simulink model "halozat_4_szet"  (R2013a)
settings: Solver=ode23s  StartTime=0.0  StopTime=5  MaxStep=0.0001  RelTol=1e-4
InitFcn:
  | punct
undefined symbols (not defined in the file or in its folder): get, Ion, Lithium
libraries: powerlib x79, simulink x37, dspsigops x18, powerlib_extras x4, dspsnks4 x2, dsparch4 x2, dspxfrm3 x1, commsequence2 x1, electricdrivelib x1
settings Model: ExtModeAutoUpdateStatusClock=off  Creator=gorbep  LastModifiedBy=Neukirchner László
settings SolverCC: PositivePriorityOrder=on
settings DataIOCC: SignalLoggingSaveFormat=ModelDataLogs
settings OptimizationCC: ExpressionDepthLimit=2147483647  InitFltsAndDblsToZero=on
settings DebuggingCC: MultiTaskDSMMsg=warning  MultiTaskCondExecSysMsg=none  FcnCallInpInsideContextMsg=UseLocalSettings  StrictBusMsg=None
settings RTWCC: IncludeERTFirstTime=on
settings GRTTargetCC: CodeReplacementLibrary=None  CombineOutputUpdateFcns=off  CPPClassGenCompliant=on  GRTInterface=on

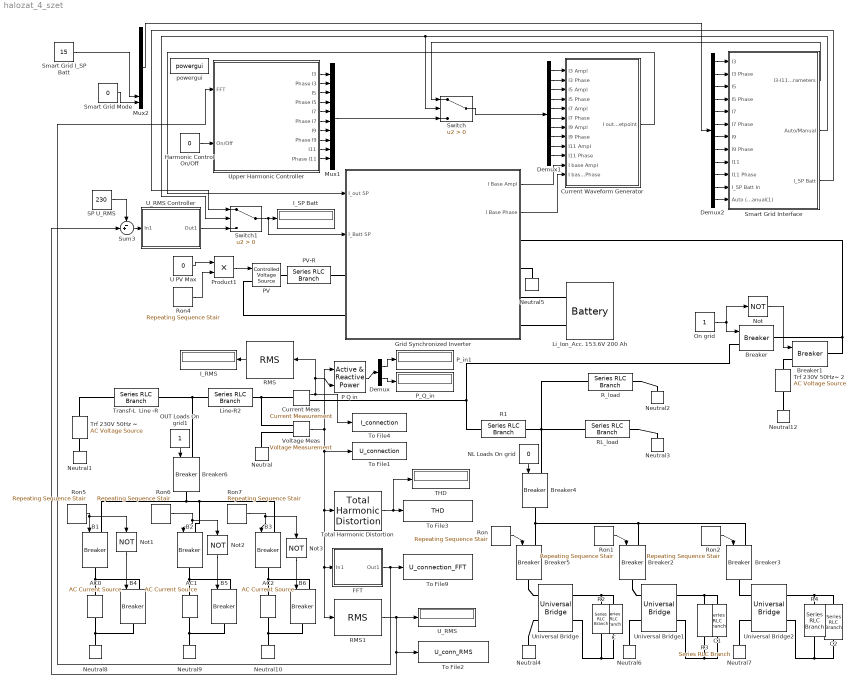
== system halozat_4_szet ==
  AC0 : powerlib/Electrical Sources/AC Current Source  Amplitude=-50  Phase=0  Frequency=50  SampleTime=0  Measurements=None
  AC1 : powerlib/Electrical Sources/AC Current Source  Amplitude=20  Phase=0  Frequency=50  SampleTime=0  Measurements=None
  AC2 : powerlib/Electrical Sources/AC Current Source  Amplitude=-30  Phase=0  Frequency=50  SampleTime=0  Measurements=None
  B{1..6} (6 alike) : powerlib/Elements/Breaker  BreakerResistance=0.01  InitialState=0  SnubberResistance=1e7  SnubberCapacitance=inf  SwitchingTimes="[ 1/60  5/60 ]"  External=on  Measurements=None  MoreParameters=off  NoBreakLoop=off
  Breaker{,1..6} (7 alike) : powerlib/Elements/Breaker  BreakerResistance=0.01  InitialState=0  SnubberResistance=1e7  SnubberCapacitance=inf  SwitchingTimes="[ 1/60  5/60 ]"  External=on  Measurements=None  MoreParameters=off  NoBreakLoop=off
  C : powerlib/Elements/Series RLC Branch  LConnTagsString=__new0  RConnTagsString=__new0  BranchType=C  Resistance=35.35  Inductance=0.1125  SetiL0=off  InitialCurrent=0  Capacitance=10e-3  Setx0=off  InitialVoltage=0  Measurements=None
  C1 : powerlib/Elements/Series RLC Branch  LConnTagsString=__new0  RConnTagsString=__new0  BranchType=C  Resistance=35.35  Inductance=0.1125  SetiL0=off  InitialCurrent=0  Capacitance=5e-3  Setx0=off  InitialVoltage=0  Measurements=None
  C2 : powerlib/Elements/Series RLC Branch  LConnTagsString=__new0  RConnTagsString=__new0  BranchType=C  Resistance=35.35  Inductance=0.1125  SetiL0=off  InitialCurrent=0  Capacitance=7e-3  Setx0=off  InitialVoltage=0  Measurements=None
  Current Meas : powerlib/Measurements/Current Measurement  PhasorSimulation=off  OutputType=Complex  PSBequivalent=0
  Current Waveform Generator : Subsystem
  Demux : Demux  Outputs=2
  Demux1 : Demux  Outputs=10
  Demux2 : Demux  Outputs=12
  FFT : Subsystem
  Grid Synchronized Inverter : Subsystem
  Harmonic Control On/Off : Constant  Value=0
  I_RMS : Display
  I_SP Batt : Display
  Li_Ion_Acc. 153.6V 200 Ah : electricdrivelib/Extra Sources/Battery  BatType=Lithium-Ion  ShowDetailedParameters=off  NomV=153.6  NomQ=200  SOC=100  PresetModel=off  MaxQ=210  FullV=274.6189824  Dis_rate=173.913  R=0.00768  Normal_OP=361.7392  expZone=[254.8950528 19.652174]  Dis_Char=off  current=[1.5 3]  Units=Ampere-hour  Batt_Tr=30
  Line-R2 : powerlib/Elements/Series RLC Branch  LConnTagsString=__new0  RConnTagsString=__new0  BranchType=R  Resistance=0.1  Inductance=0.003185  SetiL0=off  InitialCurrent=0  Capacitance=1.0  Setx0=off  InitialVoltage=0  Measurements=None
  Mux1 : Mux  Inputs=10
  Mux2 : Mux  Inputs=12
  NL Loads On grid : Constant  Value=0
  Neutral{,1..10,12} (12 alike) : powerlib/Elements/Neutral  LConnTagsString=a  NodeNumber=10
  Not{,1..3} (4 alike) : Logic  Operator=NOT  IconShape=distinctive  AllPortsSameDT=off  OutDataTypeStr=boolean
  OUT Loads On grid1 : Constant
  On grid : Constant
  P Q in : powerlib_extras/Measurements/Active & Reactive Power  f1=50
  PV : powerlib/Electrical Sources/Controlled Voltage Source  Initialize=off  Source_Type=AC  Amplitude=0  Phase=0  Frequency=0  Measurements=None
  PV-R : powerlib/Elements/Series RLC Branch  LConnTagsString=__new0  RConnTagsString=__new0  BranchType=R  Resistance=5  Inductance=0.1  SetiL0=off  InitialCurrent=0  Capacitance=1.0  Setx0=off  InitialVoltage=0  Measurements=None
  P_Q_in : Display
  P_in1 : Display
  Product1 : Product  RndMeth=Zero
  R1 : powerlib/Elements/Series RLC Branch  LConnTagsString=__new0  RConnTagsString=__new0  BranchType=R  Resistance=0.2  Inductance=0.003185  SetiL0=off  InitialCurrent=0  Capacitance=1.0  Setx0=off  InitialVoltage=0  Measurements=None
  R2 : powerlib/Elements/Series RLC Branch  LConnTagsString=__new0  RConnTagsString=__new0  BranchType=R  Resistance=25  Inductance=0.003185  SetiL0=off  InitialCurrent=0  Capacitance=1.0  Setx0=off  InitialVoltage=0  Measurements=None
  R3 : powerlib/Elements/Series RLC Branch  LConnTagsString=__new0  RConnTagsString=__new0  BranchType=R  Resistance=50  Inductance=0.003185  SetiL0=off  InitialCurrent=0  Capacitance=1.0  Setx0=off  InitialVoltage=0  Measurements=None
  R4 : powerlib/Elements/Series RLC Branch  LConnTagsString=__new0  RConnTagsString=__new0  BranchType=R  Resistance=35  Inductance=0.003185  SetiL0=off  InitialCurrent=0  Capacitance=1.0  Setx0=off  InitialVoltage=0  Measurements=None
  RL_load : powerlib/Elements/Series RLC Branch  LConnTagsString=__new0  RConnTagsString=__new0  BranchType=RL  Resistance=35.35  Inductance=0.1125  SetiL0=off  InitialCurrent=0  Capacitance=1.0  Setx0=off  InitialVoltage=0  Measurements=None
  RMS : powerlib_extras/Measurements/RMS  f1=50
  RMS1 : powerlib_extras/Measurements/RMS  f1=50
  R_load : powerlib/Elements/Series RLC Branch  LConnTagsString=__new0  RConnTagsString=__new0  BranchType=R  Resistance=50  Inductance=0.003185  SetiL0=off  InitialCurrent=0  Capacitance=1.0  Setx0=off  InitialVoltage=0  Measurements=None
  Ron : simulink/Sources/Repeating Sequence Stair  OutValues=[1 1 0 0 0 0 0 0 0 0].'  tsamp=10  OutMin=[]  OutMax=[]  OutDataTypeStr=float('double')  OutputDataTypeScalingMode=Specify via dialog  OutDataType=float('double')  ConRadixGroup=Best Precision: Vector-wise  OutScaling=2^-12
  Ron1 : simulink/Sources/Repeating Sequence Stair  OutValues=[0 0 0 1 1 0 0 0 0 0].'  tsamp=10  OutMin=[]  OutMax=[]  OutDataTypeStr=float('double')  OutputDataTypeScalingMode=Specify via dialog  OutDataType=float('double')  ConRadixGroup=Best Precision: Vector-wise  OutScaling=2^-12
  Ron2 : simulink/Sources/Repeating Sequence Stair  OutValues=[0 0 0 0 1 0 0 0 0 0].'  tsamp=10  OutMin=[]  OutMax=[]  OutDataTypeStr=float('double')  OutputDataTypeScalingMode=Specify via dialog  OutDataType=float('double')  ConRadixGroup=Best Precision: Vector-wise  OutScaling=2^-12
  Ron4 : simulink/Sources/Repeating Sequence Stair  OutValues=[1 1 0 0].'  tsamp=0.5  OutMin=[]  OutMax=[]  OutDataTypeStr=float('double')  OutputDataTypeScalingMode=Specify via dialog  OutDataType=float('double')  ConRadixGroup=Best Precision: Vector-wise  OutScaling=2^-12
  Ron5 : simulink/Sources/Repeating Sequence Stair  OutValues=[0 1 0 0 0 0 0 0 0 0].'  tsamp=1  OutMin=[]  OutMax=[]  OutDataTypeStr=float('double')  OutputDataTypeScalingMode=Specify via dialog  OutDataType=float('double')  ConRadixGroup=Best Precision: Vector-wise  OutScaling=2^-12
  Ron6 : simulink/Sources/Repeating Sequence Stair  OutValues="[0 0 0  1 0 0 0 0 0 0].'"  tsamp=1  OutMin=[]  OutMax=[]  OutDataTypeStr=float('double')  OutputDataTypeScalingMode=Specify via dialog  OutDataType=float('double')  ConRadixGroup=Best Precision: Vector-wise  OutScaling=2^-12
  Ron7 : simulink/Sources/Repeating Sequence Stair  OutValues=[0 0 0 0 1 0 0 0 0 0].'  tsamp=1  OutMin=[]  OutMax=[]  OutDataTypeStr=float('double')  OutputDataTypeScalingMode=Specify via dialog  OutDataType=float('double')  ConRadixGroup=Best Precision: Vector-wise  OutScaling=2^-12
  SP U_RMS : Constant  Value=230
  Smart Grid I_SP Batt : Constant  Value=15
  Smart Grid Mode : Constant  Value=0
  Smart Grid Interface : Subsystem
  Sum3 : Sum  Inputs=-+|
  Switch : Switch  Criteria=u2 > Threshold
  Switch1 : Switch  Criteria=u2 > Threshold
  THD : Display
  To File1 : ToFile  Filename=U_connection  MatrixName=y  SampleTime=5e-5
  To File2 : ToFile  Filename=U_conn_RMS  MatrixName=y  SampleTime=1e-3
  To File3 : ToFile  Filename=THD  MatrixName=y  SampleTime=1e-3
  To File4 : ToFile  Filename=I_connection  MatrixName=y  SampleTime=5e-5
  To File9 : ToFile  Filename=U_connection_FFT  MatrixName=y  SampleTime=1e-3
  Total Harmonic Distortion : powerlib_extras/Measurements/Total Harmonic Distortion  f1=50
  Transf-L  Line -R : powerlib/Elements/Series RLC Branch  LConnTagsString=__new0  RConnTagsString=__new0  BranchType=RL  Resistance=0.4  Inductance=0.003185  SetiL0=off  InitialCurrent=0  Capacitance=1.0  Setx0=off  InitialVoltage=0  Measurements=None
  Trf 230V 50Hz ~ : powerlib/Electrical Sources/AC Voltage Source  Amplitude=325.2691  Phase=0  Frequency=50  SampleTime=0  Measurements=None
  Trf 230V 50Hz~ 2 : powerlib/Electrical Sources/AC Voltage Source  Amplitude=325.2691  Phase=0  Frequency=50  SampleTime=0  Measurements=None
  U PV Max : Constant  Value=0
  U_RMS : Display
  U_RMS Controller : Subsystem
  Universal Bridge : powerlib/Power Electronics/Universal Bridge  Arms=2  SnubberResistance=1e5  SnubberCapacitance=inf  Device=Diodes  Ron=1e-3  Lon=0  ForwardVoltages="[  0  0  ]"  ForwardVoltage=0.8  GTOparameters=[ 10e-6 , 20e-6 ]  IGBTparameters=[ 1e-6 , 2e-6 ]  Measurements=None  Measurements_2=None  converterType=Rectifier
  Universal Bridge1 : powerlib/Power Electronics/Universal Bridge  Arms=2  SnubberResistance=1e5  SnubberCapacitance=inf  Device=Diodes  Ron=1e-3  Lon=0  ForwardVoltages="[  0  0  ]"  ForwardVoltage=0.8  GTOparameters=[ 10e-6 , 20e-6 ]  IGBTparameters=[ 1e-6 , 2e-6 ]  Measurements=None  Measurements_2=None  converterType=Rectifier
  Universal Bridge2 : powerlib/Power Electronics/Universal Bridge  Arms=2  SnubberResistance=1e5  SnubberCapacitance=inf  Device=Diodes  Ron=1e-3  Lon=0  ForwardVoltages="[  0  0  ]"  ForwardVoltage=0.8  GTOparameters=[ 10e-6 , 20e-6 ]  IGBTparameters=[ 1e-6 , 2e-6 ]  Measurements=None  Measurements_2=None  converterType=Rectifier
  Upper Harmonic Controller : Subsystem
  Voltage Meas : powerlib/Measurements/Voltage Measurement  PhasorSimulation=off  OutputType=Complex  PSBequivalent=0
  powergui : powerlib/powergui  SimulationMode=Continuous  SolverType=Tustin  SampleTime=50e-6  frequency=60  SPID=off  DisableSnubberDevices=off  DisableRonSwitches=off  DisableVfSwitches=off  SwTol=0  Interpol=off  DisplayEquations=off  frequencyindice=50  Pbase=100e6  ErrMax=1e-4  Iterations=50  UnitsV=kV  UnitsW=MW  FunctionMessages=off  echomessages=off  HookPort=off  EnableUseOfTLC=off  x0status=blocks  RestoreLinks=warning  ResistiveCurrentMeasurement=off  Frange=[0:2:500]  Ylog=off  Xlog=on  ShowGrid=off  save=off  variable=ZData  structure=0  ZoomFFT=on  StartTime=0.0  cycles=1  DisplayStyle=1  fundamental=60  FreqAxis=off  MaxFrequency=1000  frequencyindicesteady=1  RmsSteady=1  display=off  Ts=0  methode=off
  wires:
  Voltage Meas/1 -> To File1/1, Total Harmonic Distortion/1, RMS1/1, FFT/1(In1), P Q in/1
  Current Meas/1 -> To File4/1, RMS/1, P Q in/2
  On grid/1 -> Breaker/1, Not/1
  Not/1 -> Breaker1/1
  Total Harmonic Distortion/1 -> THD/1, To File3/1
  Harmonic Control On/Off/1 -> Upper Harmonic Controller/2(On/Off)
  FFT/1(Out1) -> Upper Harmonic Controller/1(FFT), To File9/1
  Ron1/1 -> Breaker2/1
  Grid Synchronized Inverter/2(I Base Phase) -> Current Waveform Generator/12(I base Phase)
  Current Waveform Generator/1(I out Setpoint) -> Grid Synchronized Inverter/1(I_out SP)
  Ron/1 -> Breaker5/1
  RMS/1 -> I_RMS/1
  Demux/1 -> P_in1/1
  P Q in/1 -> Demux/1
  Demux/2 -> P_Q_in/1
  Product1/1 -> PV/1
  U PV Max/1 -> Product1/1
  Ron4/1 -> Product1/2
  RMS1/1 -> U_RMS/1, Sum3/2, To File2/1
  Ron2/1 -> Breaker3/1
  NL Loads On grid/1 -> Breaker4/1
  OUT Loads On grid1/1 -> Breaker6/1
  Sum3/1 -> U_RMS Controller/1(In1)
  SP U_RMS/1 -> Sum3/1
  Ron5/1 -> B1/1, Not1/1
  Ron6/1 -> B2/1, Not2/1
  Ron7/1 -> B3/1, Not3/1
  Not1/1 -> B4/1
  Not2/1 -> B5/1
  Not3/1 -> B6/1
  Upper Harmonic Controller/1(I3) -> Mux1/1
  Upper Harmonic Controller/2(Phase I3) -> Mux1/2
  Upper Harmonic Controller/3(I5) -> Mux1/3
  Upper Harmonic Controller/4(Phase I5) -> Mux1/4
  Upper Harmonic Controller/5(I7) -> Mux1/5
  Upper Harmonic Controller/6(Phase I7) -> Mux1/6
  Upper Harmonic Controller/7(I9) -> Mux1/7
  Upper Harmonic Controller/8(Phase I9) -> Mux1/8
  Upper Harmonic Controller/9(I11) -> Mux1/9
  Upper Harmonic Controller/10(Phase I11) -> Mux1/10
  Demux1/1 -> Current Waveform Generator/1(I3 Ampl)
  Demux1/2 -> Current Waveform Generator/2(I3 Phase)
  Demux1/3 -> Current Waveform Generator/3(I5 Ampl)
  Demux1/4 -> Current Waveform Generator/4(I5 Phase)
  Demux1/5 -> Current Waveform Generator/5(I7 Ampl)
  Demux1/6 -> Current Waveform Generator/6(I7 Phase)
  Demux1/7 -> Current Waveform Generator/7(I9 Ampl)
  Demux1/8 -> Current Waveform Generator/8(I9 Phase)
  Demux1/9 -> Current Waveform Generator/9(I11 Ampl)
  Demux1/10 -> Current Waveform Generator/10(I11 Phase)
  Switch/1 -> Demux1/1
  Mux1/1 -> Switch/3
  Smart Grid Interface/1(I3-I11 Parameters) -> Switch/1
  Smart Grid Interface/2(Auto/Manual) -> Switch/2, Switch1/2
  U_RMS Controller/1(Out1) -> Switch1/3
  Switch1/1 -> I_SP Batt/1, Grid Synchronized Inverter/2(I_Batt SP)
  Smart Grid Interface/3(I_SP Batt) -> Switch1/1
  Grid Synchronized Inverter/1(I Base Ampl) -> Current Waveform Generator/11(I base Ampl)
  Demux2/1 -> Smart Grid Interface/1(I3)
  Demux2/2 -> Smart Grid Interface/2(I3 Phase)
  Demux2/3 -> Smart Grid Interface/3(I5)
  Demux2/4 -> Smart Grid Interface/4(I5 Phase)
  Demux2/5 -> Smart Grid Interface/5(I7)
  Demux2/6 -> Smart Grid Interface/6(I7 Phase)
  Demux2/7 -> Smart Grid Interface/7(I9)
  Demux2/8 -> Smart Grid Interface/8(I9 Phase)
  Demux2/9 -> Smart Grid Interface/9(I11)
  Demux2/10 -> Smart Grid Interface/10(I11 Phase)
  Demux2/11 -> Smart Grid Interface/11(I_SP Batt In)
  Demux2/12 -> Smart Grid Interface/12(Auto (0) / Manual(1))
  Mux2/1 -> Demux2/1
  Smart Grid Mode/1 -> Mux2/12
  Smart Grid I_SP Batt/1 -> Mux2/11
  connections:
  Trf 230V 50Hz ~/LConn1 -- Neutral1/LConn1
  Transf-L  Line -R/LConn1 -- Trf 230V 50Hz ~/RConn1
  Voltage Meas/LConn1 -- Current Meas/LConn1 -- Line-R2/RConn1
  Neutral/LConn1 -- Voltage Meas/LConn2
  Current Meas/RConn1 -- R1/LConn1 -- Breaker/LConn1
  R_load/RConn1 -- Neutral2/LConn1
  RL_load/RConn1 -- Neutral3/LConn1
  Neutral4/LConn1 -- Universal Bridge/LConn2
  Trf 230V 50Hz~ 2/LConn1 -- Neutral12/LConn1
  Grid Synchronized Inverter/RConn1 -- Breaker1/RConn1 -- Breaker/RConn1
  Breaker2/LConn1 -- Breaker3/LConn1 -- Breaker5/LConn1 -- Breaker4/RConn1
  Breaker1/LConn1 -- Trf 230V 50Hz~ 2/RConn1
  Breaker5/RConn1 -- Universal Bridge/LConn1
  C/LConn1 -- Universal Bridge/RConn1 -- R2/LConn1
  C/RConn1 -- Universal Bridge/RConn2 -- R2/RConn1
  Universal Bridge1/RConn1 -- C1/LConn1 -- R3/LConn1
  Breaker2/RConn1 -- Universal Bridge1/LConn1
  Neutral6/LConn1 -- Universal Bridge1/LConn2
  PV/RConn1 -- PV-R/LConn1
  PV/LConn1 -- Grid Synchronized Inverter/LConn2
  PV-R/RConn1 -- Grid Synchronized Inverter/LConn1
  Neutral5/LConn1 -- Grid Synchronized Inverter/RConn2
  Universal Bridge1/RConn2 -- C1/RConn1 -- R3/RConn1
  Grid Synchronized Inverter/RConn3 -- Li_Ion_Acc. 153.6V 200 Ah/LConn1
  Grid Synchronized Inverter/RConn4 -- Li_Ion_Acc. 153.6V 200 Ah/LConn2
  Line-R2/LConn1 -- Transf-L  Line -R/RConn1 -- Breaker6/LConn1
  R4/LConn1 -- Universal Bridge2/RConn1 -- C2/LConn1
  R4/RConn1 -- Universal Bridge2/RConn2 -- C2/RConn1
  Breaker3/RConn1 -- Universal Bridge2/LConn1
  Neutral7/LConn1 -- Universal Bridge2/LConn2
  AC0/LConn1 -- Neutral8/LConn1 -- B4/RConn1
  B1/RConn1 -- AC0/RConn1 -- B4/LConn1
  B2/RConn1 -- AC1/RConn1 -- B5/LConn1
  AC1/LConn1 -- Neutral9/LConn1 -- B5/RConn1
  B3/RConn1 -- AC2/RConn1 -- B6/LConn1
  AC2/LConn1 -- Neutral10/LConn1 -- B6/RConn1
  R1/RConn1 -- RL_load/LConn1 -- R_load/LConn1 -- Breaker4/LConn1
  B2/LConn1 -- B3/LConn1 -- B1/LConn1 -- Breaker6/RConn1

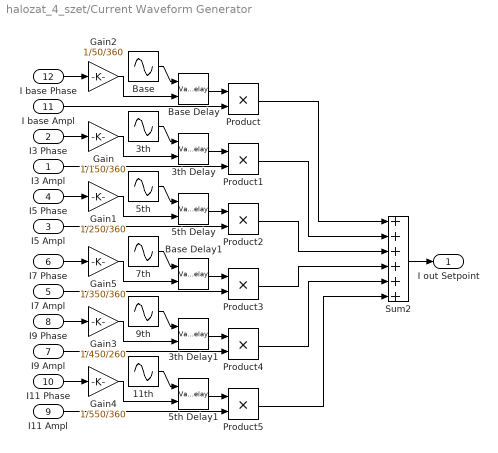
== system halozat_4_szet/Current Waveform Generator ==
  I3 Ampl : Inport
  I3 Phase : Inport  Port=2
  I5 Ampl : Inport  Port=3
  I5 Phase : Inport  Port=4
  I7 Ampl : Inport  Port=5
  I7 Phase : Inport  Port=6
  I9 Ampl : Inport  Port=7
  I9 Phase : Inport  Port=8
  I11 Ampl : Inport  Port=9
  I11 Phase : Inport  Port=10
  I base Ampl : Inport  Port=11
  I base Phase : Inport  Port=12
  11th : Sin  Frequency=110*pi  SampleTime=0
  3th : Sin  Frequency=300*pi  SampleTime=0
  3th Delay : VariableTransportDelay  MaximumDelay=10  ZeroDelay=on
  3th Delay1 : VariableTransportDelay  MaximumDelay=10  ZeroDelay=on
  5th : Sin  Frequency=500*pi  SampleTime=0
  5th Delay : VariableTransportDelay  MaximumDelay=10  ZeroDelay=on
  5th Delay1 : VariableTransportDelay  MaximumDelay=10  ZeroDelay=on
  7th : Sin  Frequency=700*pi  SampleTime=0
  9th : Sin  Frequency=900*pi  SampleTime=0
  Base : Sin  Frequency=100*pi  SampleTime=0
  Base Delay : VariableTransportDelay  MaximumDelay=10  ZeroDelay=on
  Base Delay1 : VariableTransportDelay  MaximumDelay=10  ZeroDelay=on
  Gain : Gain  Gain=1/150/360
  Gain1 : Gain  Gain=1/250/360
  Gain2 : Gain  Gain=1/50/360
  Gain3 : Gain  Gain=1/450/260
  Gain4 : Gain  Gain=1/550/360
  Gain5 : Gain  Gain=1/350/360
  Product{,1..5} (6 alike) : Product  RndMeth=Zero
  Sum2 : Sum  Inputs=++++++
  I out Setpoint : Outport
  wires:
  Base/1 -> Base Delay/1
  Base Delay/1 -> Product/1
  3th Delay/1 -> Product1/1
  5th Delay/1 -> Product2/1
  3th/1 -> 3th Delay/1
  5th/1 -> 5th Delay/1
  Gain/1 -> 3th Delay/2
  Gain1/1 -> 5th Delay/2
  Gain2/1 -> Base Delay/2
  I base Ampl/1 -> Product/2
  I base Phase/1 -> Gain2/1
  I3 Phase/1 -> Gain/1
  Sum2/1 -> I out Setpoint/1
  I3 Ampl/1 -> Product1/2
  I5 Phase/1 -> Gain1/1
  I5 Ampl/1 -> Product2/2
  7th/1 -> Base Delay1/1
  Base Delay1/1 -> Product3/1
  3th Delay1/1 -> Product4/1
  5th Delay1/1 -> Product5/1
  9th/1 -> 3th Delay1/1
  11th/1 -> 5th Delay1/1
  Gain3/1 -> 3th Delay1/2
  Gain4/1 -> 5th Delay1/2
  Gain5/1 -> Base Delay1/2
  I7 Ampl/1 -> Product3/2
  I7 Phase/1 -> Gain5/1
  I9 Phase/1 -> Gain3/1
  I9 Ampl/1 -> Product4/2
  I11 Phase/1 -> Gain4/1
  I11 Ampl/1 -> Product5/2
  Product/1 -> Sum2/1
  Product1/1 -> Sum2/2
  Product2/1 -> Sum2/3
  Product3/1 -> Sum2/4
  Product4/1 -> Sum2/5
  Product5/1 -> Sum2/6

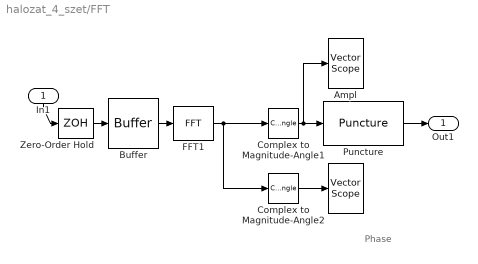
== system halozat_4_szet/FFT ==
  note: Phase
  In1 : Inport
  " " : dspsnks4/Vector Scope  ScopeProperties=off  Domain=Frequency  HorizSpan=1  DisplayProperties=off  AxisGrid=on  Memory=off  FrameNumber=on  AxisLegend=off  AxisZoom=off  OpenScopeAtSimStart=on  OpenScopeImmediately=off  FigPos=get(0,'defaultfigureposition')  AxisProperties=on  XUnits=Hertz  XRange=[0...Fs/2]  InheritXIncr=on  XIncr=0.001  XLabel=Samples  XLimit=Auto  XMin=0  XMax=1  XStart=0  YUnits=Magnitude  YLabel=Amplitude  LineProperties=off  XAxisParamsVer=6.9
      settings: YMin=0  YMax=12
  Ampl : dspsnks4/Vector Scope  ScopeProperties=off  Domain=Frequency  HorizSpan=1  DisplayProperties=off  AxisGrid=on  Memory=off  FrameNumber=on  AxisLegend=off  AxisZoom=off  OpenScopeAtSimStart=on  OpenScopeImmediately=off  FigPos=get(0,'defaultfigureposition')  AxisProperties=on  XUnits=Hertz  XRange=[0...Fs/2]  InheritXIncr=on  XIncr=0.001  XLabel=Samples  XLimit=Auto  XMin=0  XMax=1  XStart=0  YUnits=Magnitude  YLabel=Amplitude  LineProperties=off  XAxisParamsVer=6.8
      settings: YMin=0  YMax=12
  Buffer : Buffer  N=128
  Complex to Magnitude-Angle1 : ComplexToMagnitudeAngle  Output=Magnitude
  Complex to Magnitude-Angle2 : ComplexToMagnitudeAngle  Output=Angle
  FFT1 : dspxfrm3/FFT  CompMethod=Table lookup  TableOpt=HYBRID  TableOptActive=Speed  BitRevOrder=off  InheritFFTLength=on  FFTLength=64  RowConvenienceOn=on  FFTImplementation=Auto  SkipNorm=on  firstCoeffDataTypeStr=Inherit: Same word length as input  firstCoeffLastDataTypeStr=Inherit: Same word length as input  outputMin=[]  outputMax=[]  roundingMode=Floor  overflowMode=off
  Puncture : commsequence2/Puncture  punctureVector=s'
  Zero-Order Hold : ZeroOrderHold  SampleTime=20e-3/128
  Out1 : Outport
  wires:
  FFT1/1 -> Complex to Magnitude-Angle1/1, Complex to Magnitude-Angle2/1
  Buffer/1 -> FFT1/1
  Zero-Order Hold/1 -> Buffer/1
  Complex to Magnitude-Angle1/1 -> Puncture/1, Ampl/1
  In1/1 -> Zero-Order Hold/1
  Puncture/1 -> Out1/1
  Complex to Magnitude-Angle2/1 -> " "/1

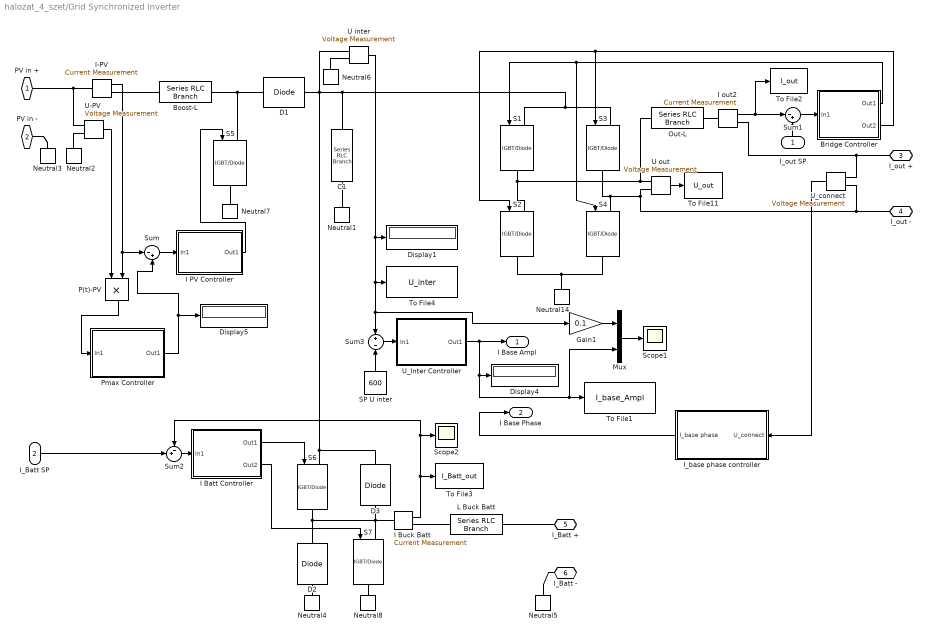
== system halozat_4_szet/Grid Synchronized Inverter ==
  I_out SP : Inport
  I_Batt SP : Inport  Port=2
  " Boost-L" : powerlib/Elements/Series RLC Branch  LConnTagsString=__new0  RConnTagsString=__new0  BranchType=L  Resistance=8  Inductance=100e-3  SetiL0=off  InitialCurrent=30  Capacitance=1.0  Setx0=off  InitialVoltage=0  Measurements=None
  " Out-L" : powerlib/Elements/Series RLC Branch  LConnTagsString=__new0  RConnTagsString=__new0  BranchType=L  Resistance=100  Inductance=10e-3  SetiL0=off  InitialCurrent=0  Capacitance=1.0  Setx0=off  InitialVoltage=0  Measurements=None
  Bridge Controller : Subsystem
  C1 : powerlib/Elements/Series RLC Branch  LConnTagsString=__new0  RConnTagsString=__new0  BranchType=C  Resistance=35.35  Inductance=0.1125  SetiL0=off  InitialCurrent=0  Capacitance=10e-3  Setx0=on  InitialVoltage=600  Measurements=None
  D1 : powerlib/Power Electronics/Diode  Ron=0.001  Lon=0  Vf=0.8  IC=0  UseSnubber=off  Rs=50000  Cs=250e-9  Measurements=off
  D2 : powerlib/Power Electronics/Diode  Ron=0.001  Lon=0  Vf=0.8  IC=0  UseSnubber=off  Rs=50000  Cs=250e-9  Measurements=off
  D3 : powerlib/Power Electronics/Diode  Ron=0.001  Lon=0  Vf=0.8  IC=0  UseSnubber=off  Rs=50000  Cs=250e-9  Measurements=off
  Display1 : Display
  Display4 : Display
  Display5 : Display
  Gain1 : Gain  Gain=0.1
  I Batt Controller : Subsystem
  I Buck Batt : powerlib/Measurements/Current Measurement  PhasorSimulation=off  OutputType=Complex  PSBequivalent=0
  I PV Controller : Subsystem
  I out2 : powerlib/Measurements/Current Measurement  PhasorSimulation=off  OutputType=Complex  PSBequivalent=0
  I-PV : powerlib/Measurements/Current Measurement  PhasorSimulation=off  OutputType=Complex  PSBequivalent=0
  I_base phase controller : Subsystem
  L Buck Batt : powerlib/Elements/Series RLC Branch  LConnTagsString=__new0  RConnTagsString=__new0  BranchType=L  Resistance=100  Inductance=1e-1  SetiL0=on  InitialCurrent=0  Capacitance=1.0  Setx0=off  InitialVoltage=0  Measurements=None
  Mux : Mux  Inputs=2
  Neutral{1..8,14} (9 alike) : powerlib/Elements/Neutral  LConnTagsString=a  NodeNumber=1
  P(t)-PV : Product  RndMeth=Zero
  Pmax Controller : Subsystem
  S{1..7} (7 alike) : powerlib/Power Electronics/IGBT//Diode  Ron=1e-3  Rs=1e5  Cs=inf  Measurements=off
  SP U inter : Constant  Value=600
  Scope1 : Scope
      settings: TimeRange=2  YMin=-50  YMax=70  SaveName=ScopeData4
  Scope2 : Scope
      settings: TimeRange=0.1  YMin=-40  YMax=40  SaveName=ScopeData2
  Sum : Sum  Inputs=|-+
  Sum1 : Sum  Inputs=|-+
  Sum2 : Sum  Inputs=-+|
  Sum3 : Sum  Inputs=+-
  To File1 : ToFile  Filename=I_base_Ampl  MatrixName=y  SampleTime=5e-3
  To File11 : ToFile  Filename=U_out  MatrixName=y  SampleTime=5e-5
  To File2 : ToFile  Filename=I_out  MatrixName=y  SampleTime=5e-5
  To File3 : ToFile  Filename=I_Batt_out  MatrixName=y  SampleTime=5e-3
  To File4 : ToFile  Filename=U_inter  MatrixName=y  SampleTime=5e-3
  U inter : powerlib/Measurements/Voltage Measurement  PhasorSimulation=off  OutputType=Complex  PSBequivalent=0
  U out : powerlib/Measurements/Voltage Measurement  PhasorSimulation=off  OutputType=Complex  PSBequivalent=0
  U-PV : powerlib/Measurements/Voltage Measurement  PhasorSimulation=off  OutputType=Complex  PSBequivalent=0
  U_Inter Controller : Subsystem
  U_connect : powerlib/Measurements/Voltage Measurement  PhasorSimulation=off  OutputType=Complex  PSBequivalent=0
  " PV in +" : PMIOPort  Port=1  Side=Left
  " PV in -" : PMIOPort  Port=2  Side=Left
  " I_out +" : PMIOPort  Port=3  Side=Right
  " I_out -" : PMIOPort  Port=4  Side=Right
  " I_Batt +" : PMIOPort  Port=5  Side=Right
  " I_Batt -" : PMIOPort  Port=6  Side=Right
  I Base Ampl : Outport
  I Base Phase : Outport  Port=2
  wires:
  U inter/1 -> Display1/1, Sum3/1, Gain1/1, To File4/1
  Sum/1 -> I PV Controller/1(In1)
  I-PV/1 -> Sum/1, P(t)-PV/2
  I out2/1 -> Sum1/1, To File2/1
  Bridge Controller/2(Out2) -> S3/1, S2/1
  Bridge Controller/1(Out1) -> S1/1, S4/1
  SP U inter/1 -> Sum3/2
  U-PV/1 -> P(t)-PV/1
  Pmax Controller/1(Out1) -> Display5/1, Sum/2
  I PV Controller/1(Out1) -> S5/1
  Sum1/1 -> Bridge Controller/1(In1)
  P(t)-PV/1 -> Pmax Controller/1(In1)
  U_Inter Controller/1(Out1) -> I Base Ampl/1, To File1/1, Mux/2, Display4/1
  Sum3/1 -> U_Inter Controller/1(In1)
  U out/1 -> To File11/1
  I_out SP/1 -> Sum1/2
  Sum2/1 -> I Batt Controller/1(In1)
  I Buck Batt/1 -> To File3/1, Scope2/1, Sum2/1
  I Batt Controller/1(Out1) -> S6/1
  Mux/1 -> Scope1/1
  Gain1/1 -> Mux/1
  U_connect/1 -> I_base phase controller/1(U_connect)
  I_base phase controller/1(I_base phase) -> I Base Phase/1
  I_Batt SP/1 -> Sum2/2
  I Batt Controller/2(Out2) -> S7/1
  connections:
  " Boost-L"/RConn1 -- D1/LConn1 -- S5/LConn1
  " PV in +"/RConn1 -- I-PV/LConn1 -- U-PV/LConn1
  U out/LConn1 -- " Out-L"/LConn1 -- S2/LConn1 -- S1/RConn1
  S6/LConn1 -- U inter/LConn1 -- D1/RConn1 -- S1/LConn1 -- S3/LConn1 -- C1/LConn1 -- D3/RConn1
  S4/RConn1 -- S2/RConn1 -- Neutral14/LConn1
  U out/LConn2 -- S4/LConn1 -- S3/RConn1 -- " I_out -"/RConn1 -- U_connect/LConn2
  Neutral6/LConn1 -- U inter/LConn2
  Neutral7/LConn1 -- S5/RConn1
  I-PV/RConn1 -- " Boost-L"/LConn1
  " Out-L"/RConn1 -- I out2/LConn1
  Neutral1/LConn1 -- C1/RConn1
  U-PV/LConn2 -- Neutral2/LConn1
  " PV in -"/RConn1 -- Neutral3/LConn1
  " I_out +"/RConn1 -- I out2/RConn1 -- U_connect/LConn1
  L Buck Batt/LConn1 -- I Buck Batt/RConn1
  I Buck Batt/LConn1 -- S7/LConn1 -- D3/LConn1 -- S6/RConn1 -- D2/RConn1
  Neutral4/LConn1 -- D2/LConn1
  L Buck Batt/RConn1 -- " I_Batt +"/RConn1
  Neutral5/LConn1 -- " I_Batt -"/RConn1
  S7/RConn1 -- Neutral8/LConn1

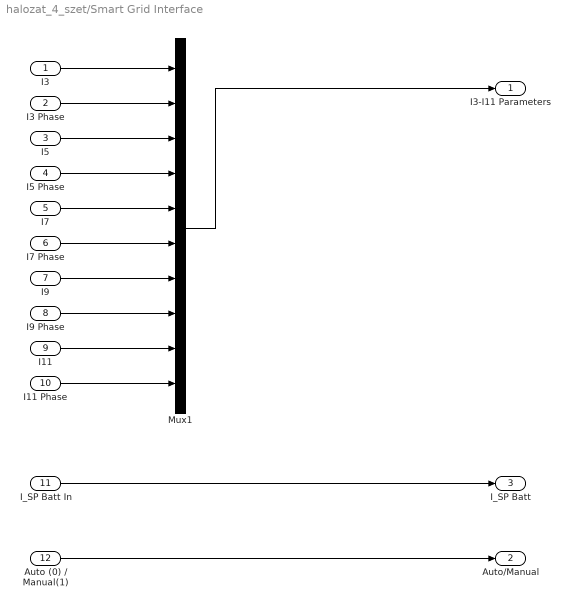
== system halozat_4_szet/Smart Grid Interface ==
  I3 : Inport
  I3 Phase : Inport  Port=2
  I5 : Inport  Port=3
  I5 Phase : Inport  Port=4
  I7 : Inport  Port=5
  I7 Phase : Inport  Port=6
  I9 : Inport  Port=7
  I9 Phase : Inport  Port=8
  I11 : Inport  Port=9
  I11 Phase : Inport  Port=10
  I_SP Batt In : Inport  Port=11
  Auto (0) / Manual(1) : Inport  Port=12
  Mux1 : Mux  Inputs=10
  I3-I11 Parameters : Outport
  Auto/Manual : Outport  Port=2
  I_SP Batt : Outport  Port=3
  wires:
  I3/1 -> Mux1/1
  I3 Phase/1 -> Mux1/2
  I5/1 -> Mux1/3
  I5 Phase/1 -> Mux1/4
  I7/1 -> Mux1/5
  I7 Phase/1 -> Mux1/6
  I9/1 -> Mux1/7
  I9 Phase/1 -> Mux1/8
  I11/1 -> Mux1/9
  I11 Phase/1 -> Mux1/10
  Mux1/1 -> I3-I11 Parameters/1
  Auto (0) / Manual(1)/1 -> Auto/Manual/1
  I_SP Batt In/1 -> I_SP Batt/1

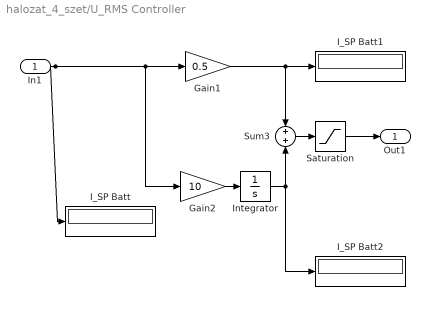
== system halozat_4_szet/U_RMS Controller ==
  In1 : Inport
  Gain1 : Gain  Gain=0.5
  Gain2 : Gain  Gain=10
  I_SP Batt : Display
  I_SP Batt1 : Display
  I_SP Batt2 : Display
  Integrator : Integrator  LimitOutput=on  UpperSaturationLimit=100  LowerSaturationLimit=-100
  Saturation : Saturate  UpperLimit=100  LowerLimit=-100
  Sum3 : Sum
  Out1 : Outport
  wires:
  Saturation/1 -> Out1/1
  In1/1 -> Gain1/1, Gain2/1, I_SP Batt/1
  Sum3/1 -> Saturation/1
  Gain1/1 -> Sum3/1, I_SP Batt1/1
  Integrator/1 -> Sum3/2, I_SP Batt2/1
  Gain2/1 -> Integrator/1

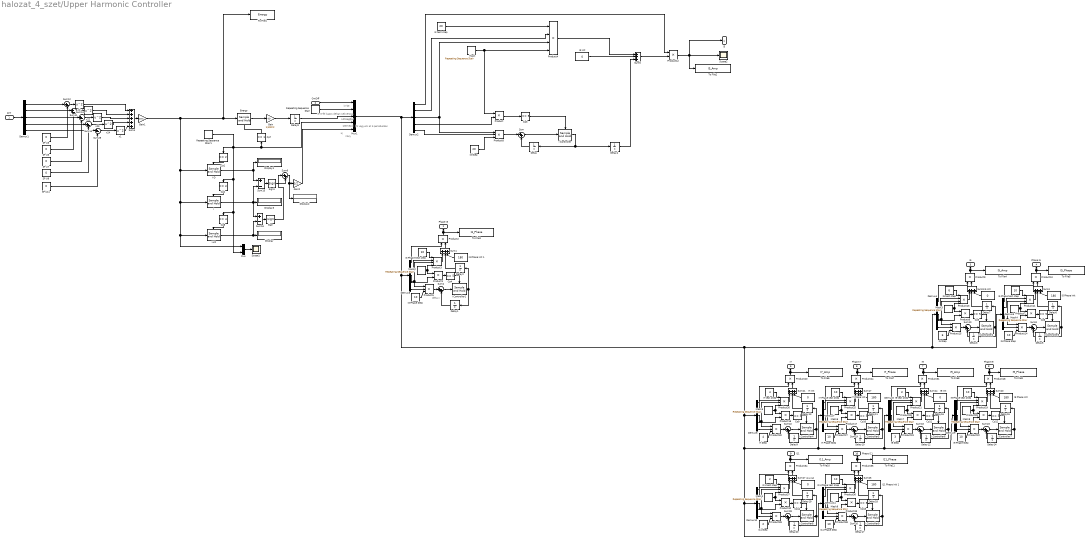
== system halozat_4_szet/Upper Harmonic Controller ==
  note: delta x
  note: hl vagyunk az 5 periódusban
  note: új
  note: le-0-fel kapcs
      | deltaX sekvencia
  note: ki-be
  note: költségfgv
  note: ütemező
  note: irány
  FFT : Inport
  On/Off : Inport  Port=2
  Cp1 : simulink/Logic and Bit Operations/Compare To Constant  relop===  const=2  OutDataTypeStr=uint8  ZeroCross=off
  Cp{3..6,9..14} (10 alike) : simulink/Logic and Bit Operations/Compare To Constant  relop===  const=5  OutDataTypeStr=uint8  ZeroCross=off
  Cp2 : simulink/Logic and Bit Operations/Compare To Constant  relop===  const=3  OutDataTypeStr=uint8  ZeroCross=off
  Cp7 : simulink/Logic and Bit Operations/Compare To Constant  relop===  const=1  OutDataTypeStr=uint8  ZeroCross=off
  Cp8 : simulink/Logic and Bit Operations/Compare To Constant  relop===  const=4  OutDataTypeStr=uint8  ZeroCross=off
  Delay{,1,3,5,9..10,12,14,17,20} (10 alike) : UnitDelay  SampleTime=0.001
  Delay{2,4,6..7,11,13,15..16,18..19} (10 alike) : UnitDelay  SampleTime=0.02
  Delay8 : UnitDelay  InitialCondition=18  SampleTime=0.02
  Demux{1..11} (11 alike) : Demux  Outputs=5
  Display{,1..3} (4 alike) : Display
  Energy : dspsigops/Sample and Hold  trig=Rising edge  initCond=18  latchinput=off
  Gain : Gain  Gain=1/100*2
  Gain1 : Gain  Gain=1e-1
  Gain2 : Gain  Gain=1/2
  I : dspsigops/Sample and Hold  trig=Rising edge  initCond=0  latchinput=off
  I Controller{,1..9} (10 alike) : dspsigops/Sample and Hold  trig=Rising edge  initCond=0  latchinput=off
  I+D : dspsigops/Sample and Hold  trig=Rising edge  initCond=0  latchinput=off
  I-D : dspsigops/Sample and Hold  trig=Rising edge  initCond=0  latchinput=off
  I11 Step : Constant  Value=2
  "I11 init " : Constant  Value=0
  I11 Phase Step : Constant  Value=10
  I11 Phase init 1 : Constant  Value=180
  I11 Phase test step : Constant  Value=10
  I11 test step : Constant  Value=2
  I3 Step : Constant  Value=20
  "I3 init " : Constant  Value=0
  I3 Phase Step : Constant  Value=10
  I3 Phase init 1 : Constant  Value=180
  I3 Phase test step : Constant  Value=10
  I3 test step : Constant  Value=20
  I5 Step : Constant  Value=6
  "I5 init " : Constant  Value=0
  I5 Phase Step : Constant  Value=10
  "I5 Phase init " : Constant  Value=180
  I5 Phase test step : Constant  Value=10
  I5 test step : Constant  Value=6
  I7 Step : Constant  Value=4
  "I7 init " : Constant  Value=0
  I7 Phase Step : Constant  Value=10
  "I7 Phase init " : Constant  Value=180
  I7 Phase test step : Constant  Value=10
  I7 test step : Constant  Value=4
  I9 Step : Constant  Value=3
  "I9 init " : Constant  Value=0
  I9 Phase Step : Constant  Value=10
  "I9 Phase init " : Constant  Value=180
  I9 Phase test step : Constant  Value=10
  I9 test step : Constant  Value=3
  Mask : simulink/Sources/Repeating Sequence Stair  OutValues=[1 0 0 0 0 0 0 0 0 0].'  tsamp=0.1  OutMin=[]  OutMax=[]  OutDataTypeStr=float('double')  OutputDataTypeScalingMode=Specify via dialog  OutDataType=float('double')  ConRadixGroup=Best Precision: Vector-wise  OutScaling=2^-12
  Mask1 : simulink/Sources/Repeating Sequence Stair  OutValues=[0 0 0 0 0 0 0 0 1 0].'  tsamp=0.1  OutMin=[]  OutMax=[]  OutDataTypeStr=float('double')  OutputDataTypeScalingMode=Specify via dialog  OutDataType=float('double')  ConRadixGroup=Best Precision: Vector-wise  OutScaling=2^-12
  Mask2 : simulink/Sources/Repeating Sequence Stair  OutValues=[0 1 0 0 0 0 0 0 0 0].'  tsamp=0.1  OutMin=[]  OutMax=[]  OutDataTypeStr=float('double')  OutputDataTypeScalingMode=Specify via dialog  OutDataType=float('double')  ConRadixGroup=Best Precision: Vector-wise  OutScaling=2^-12
  Mask3 : simulink/Sources/Repeating Sequence Stair  OutValues=[0 0 1 0 0 0 0 0 0 0].'  tsamp=0.1  OutMin=[]  OutMax=[]  OutDataTypeStr=float('double')  OutputDataTypeScalingMode=Specify via dialog  OutDataType=float('double')  ConRadixGroup=Best Precision: Vector-wise  OutScaling=2^-12
  Mask4 : simulink/Sources/Repeating Sequence Stair  OutValues=[0 0 0 1 0 0 0 0 0 0].'  tsamp=0.1  OutMin=[]  OutMax=[]  OutDataTypeStr=float('double')  OutputDataTypeScalingMode=Specify via dialog  OutDataType=float('double')  ConRadixGroup=Best Precision: Vector-wise  OutScaling=2^-12
  Mask5 : simulink/Sources/Repeating Sequence Stair  OutValues=[0 0 0 0 1 0 0 0 0 0].'  tsamp=0.1  OutMin=[]  OutMax=[]  OutDataTypeStr=float('double')  OutputDataTypeScalingMode=Specify via dialog  OutDataType=float('double')  ConRadixGroup=Best Precision: Vector-wise  OutScaling=2^-12
  Mask6 : simulink/Sources/Repeating Sequence Stair  OutValues=[0 0 0 0 0 1 0 0 0 0].'  tsamp=0.1  OutMin=[]  OutMax=[]  OutDataTypeStr=float('double')  OutputDataTypeScalingMode=Specify via dialog  OutDataType=float('double')  ConRadixGroup=Best Precision: Vector-wise  OutScaling=2^-12
  Mask7 : simulink/Sources/Repeating Sequence Stair  OutValues=[0 0 0 0 0 0 1 0 0 0].'  tsamp=0.1  OutMin=[]  OutMax=[]  OutDataTypeStr=float('double')  OutputDataTypeScalingMode=Specify via dialog  OutDataType=float('double')  ConRadixGroup=Best Precision: Vector-wise  OutScaling=2^-12
  Mask8 : simulink/Sources/Repeating Sequence Stair  OutValues=[0 0 0 0 0 0 0 1 0 0].'  tsamp=0.1  OutMin=[]  OutMax=[]  OutDataTypeStr=float('double')  OutputDataTypeScalingMode=Specify via dialog  OutDataType=float('double')  ConRadixGroup=Best Precision: Vector-wise  OutScaling=2^-12
  Mask9 : simulink/Sources/Repeating Sequence Stair  OutValues=[0 0 0 0 0 0 0 0 0 1].'  tsamp=0.1  OutMin=[]  OutMax=[]  OutDataTypeStr=float('double')  OutputDataTypeScalingMode=Specify via dialog  OutDataType=float('double')  ConRadixGroup=Best Precision: Vector-wise  OutScaling=2^-12
  Mux : Mux  Inputs=2
  Mux1 : Mux  Inputs=5
  Product{,1..2,6..7,9..10,12,16..18,20,24,28..29,31..35} (20 alike) : Product  RndMeth=Zero
  Product{3..4,11,13,19,21,25..26,36..37} (10 alike) : Product  Inputs=4  RndMeth=Zero
  Product{5,8,14..15,22..23,27,30,38..39} (10 alike) : Product  Inputs=3  RndMeth=Zero
  Repeating Sequence Stair : simulink/Sources/Repeating Sequence Stair  OutValues=[-1 0 1 0 0].'  tsamp=0.02  OutMin=[]  OutMax=[]  OutDataTypeStr=float('double')  OutputDataTypeScalingMode=Specify via dialog  OutDataType=float('double')  ConRadixGroup=Best Precision: Vector-wise  OutScaling=2^-12
  Repeating Sequence Stair1 : simulink/Sources/Repeating Sequence Stair  OutValues=[1 2 3 4 5].'  tsamp=0.02  OutMin=[]  OutMax=[]  OutDataTypeStr=float('double')  OutputDataTypeScalingMode=Specify via dialog  OutDataType=float('double')  ConRadixGroup=Best Precision: Vector-wise  OutScaling=2^-12
  SP U{3,5,7,9,11} (5 alike) : Constant  Value=0
  Scope1 : Scope
      settings: TimeRange=0.2
  Scope2 : Scope
      settings: TimeRange=0.2  YMin=-200  YMax=200
  Sign : Signum
  Sign1 : Signum
  Sum{,2,6,8,10,18..19,22..23,26,28} (11 alike) : Sum  Inputs=|++
  Sum{1,3,5,9,17,20..21,24..25,27} (10 alike) : Sum  Inputs=+++
  Sum{11..14,29} (5 alike) : Sum  Inputs=|+-
  Sum15 : Sum  Inputs=+-
  Sum16 : Sum  Inputs=+-
  Sum4 : Sum  Inputs=+++++
  To File1 : ToFile  Filename=Energy  MatrixName=y  SampleTime=0.001
  To File10 : ToFile  Filename=I11_Amp  MatrixName=y  SampleTime=0.001
  To File11 : ToFile  Filename=I11_Phase  MatrixName=y  SampleTime=0.001
  To File2 : ToFile  Filename=I3_Amp  MatrixName=y  SampleTime=0.001
  To File3 : ToFile  Filename=I3_Phase  MatrixName=y  SampleTime=0.001
  To File4 : ToFile  Filename=I5_Amp  MatrixName=y  SampleTime=0.001
  To File5 : ToFile  Filename=I5_Phase  MatrixName=y  SampleTime=0.001
  To File6 : ToFile  Filename=I7_Amp  MatrixName=y  SampleTime=0.001
  To File7 : ToFile  Filename=I7_Phase  MatrixName=y  SampleTime=0.001
  To File8 : ToFile  Filename=I9_Amp  MatrixName=y  SampleTime=0.001
  To File9 : ToFile  Filename=I9_Phase  MatrixName=y  SampleTime=0.001
  x{1..2,22..24} (5 alike) : Math  Operator=square  SaturateOnIntegerOverflow=on
  I3 : Outport
  Phase I3 : Outport  Port=2
  I5 : Outport  Port=3
  Phase I5 : Outport  Port=4
  I7 : Outport  Port=5
  Phase I7 : Outport  Port=6
  I9 : Outport  Port=7
  Phase I9 : Outport  Port=8
  I11 : Outport  Port=9
  Phase I11 : Outport  Port=10
  wires:
  Cp1/1 -> I-D/Trigger
  Sum/1 -> I Controller/1
  I Controller/1 -> Delay4/1, Delay/1
  x2/1 -> Sum4/1
  Repeating Sequence Stair1/1 -> Mux1/4, Cp7/1, Cp1/1, Cp2/1, Mux/2, Cp8/1
  Product/1 -> Cp3/1
  Cp7/1 -> Energy/Trigger
  I3 test step/1 -> Product4/1
  Energy/1 -> Gain/1
  Product12/1 -> Scope2/1, I3/1, To File2/1
  SP U5/1 -> Sum11/2
  SP U3/1 -> Sum12/2
  FFT/1 -> Demux1/1
  Demux1/1 -> Sum12/1
  Demux1/2 -> Sum11/1
  SP U7/1 -> Sum13/2
  SP U9/1 -> Sum14/2
  Demux1/3 -> Sum13/1
  Demux1/4 -> Sum14/1
  Sum12/1 -> x2/1
  Sum11/1 -> x22/1
  Sum14/1 -> x24/1
  Sum13/1 -> x23/1
  x22/1 -> Sum4/2
  Cp2/1 -> I/Trigger
  Cp8/1 -> I+D/Trigger
  Mux/1 -> Scope1/1
  Sum4/1 -> Gain1/1
  Gain1/1 -> Energy/1, To File1/1, Mux/1, I+D/1, I/1, I-D/1
  I-D/1 -> Display1/1, Sum15/1
  I/1 -> Display3/1, Sum15/2, Sum16/1
  I+D/1 -> Display/1, Sum16/2
  Sum16/1 -> Sign/1
  Sum15/1 -> Sign1/1
  Sum6/1 -> Display2/1, Gain2/1
  Sum5/1 -> Product12/2
  Product4/1 -> Sum5/1
  Mask/1 -> Product/1, Product4/4
  Cp3/1 -> I Controller/Trigger
  I3 Step/1 -> Product8/3
  Gain/1 -> Delay8/1
  Mux1/1 -> Demux3/1, Demux6/1, Demux7/1, Demux9/1, Demux8/1, Demux11/1, Demux10/1, Demux5/1, Demux4/1, Demux2/1
  Demux2/1 -> Product12/1
  On/Off/1 -> Mux1/1
  Repeating Sequence Stair/1 -> Mux1/2
  Demux2/2 -> Product4/2
  Demux2/3 -> Product4/3, Product8/1
  Demux2/4 -> Product/2
  Demux2/5 -> Product8/2
  Product5/1 -> Sum2/1
  Sum2/1 -> I Controller1/1
  Delay1/1 -> Sum2/2
  I Controller1/1 -> Delay1/1, Delay2/1
  Product1/1 -> Cp4/1
  I3 Phase test step/1 -> Product3/1
  Sum1/1 -> Product2/2
  I3 Phase init 1/1 -> Sum1/3
  Product3/1 -> Sum1/1
  Mask2/1 -> Product3/4, Product1/1
  Cp4/1 -> I Controller1/Trigger
  Delay2/1 -> Sum1/2
  I3 Phase Step/1 -> Product5/3
  Demux3/1 -> Product2/1
  Demux3/2 -> Product3/2
  Demux3/3 -> Product3/3, Product5/1
  Demux3/4 -> Product1/2
  Demux3/5 -> Product5/2
  Product15/1 -> Sum10/1
  Sum10/1 -> I Controller2/1
  Delay3/1 -> Sum10/2
  I Controller2/1 -> Delay3/1, Delay7/1
  Product6/1 -> Cp5/1
  I5 test step/1 -> Product13/1
  Sum9/1 -> Product9/2
  "I5 init "/1 -> Sum9/3
  Product13/1 -> Sum9/1
  Mask3/1 -> Product13/4, Product6/1
  Cp5/1 -> I Controller2/Trigger
  Delay7/1 -> Sum9/2
  I5 Step/1 -> Product15/3
  Demux4/1 -> Product9/1
  Demux4/2 -> Product13/2
  Demux4/3 -> Product13/3, Product15/1
  Demux4/4 -> Product6/2
  Demux4/5 -> Product15/2
  Product14/1 -> Sum8/1
  Sum8/1 -> I Controller3/1
  Delay5/1 -> Sum8/2
  I Controller3/1 -> Delay5/1, Delay6/1
  Product7/1 -> Cp6/1
  I5 Phase test step/1 -> Product11/1
  Sum3/1 -> Product10/2
  "I5 Phase init "/1 -> Sum3/3
  Product11/1 -> Sum3/1
  Mask4/1 -> Product11/4, Product7/1
  Cp6/1 -> I Controller3/Trigger
  Delay6/1 -> Sum3/2
  I5 Phase Step/1 -> Product14/3
  Demux5/1 -> Product10/1
  Demux5/2 -> Product11/2
  Demux5/3 -> Product11/3, Product14/1
  Demux5/4 -> Product7/2
  Demux5/5 -> Product14/2
  Product9/1 -> I5/1, To File4/1
  Product10/1 -> Phase I5/1, To File5/1
  Product2/1 -> Phase I3/1, To File3/1
  Product30/1 -> Sum22/1
  Sum22/1 -> I Controller4/1
  Delay9/1 -> Sum22/2
  I Controller4/1 -> Delay9/1, Delay13/1
  Product16/1 -> Cp9/1
  I7 test step/1 -> Product26/1
  Product20/1 -> I7/1, To File6/1
  Sum21/1 -> Product20/2
  "I7 init "/1 -> Sum21/3
  Product26/1 -> Sum21/1
  Mask5/1 -> Product26/4, Product16/1
  Cp9/1 -> I Controller4/Trigger
  Delay13/1 -> Sum21/2
  I7 Step/1 -> Product30/3
  Demux6/1 -> Product20/1
  Demux6/2 -> Product26/2
  Demux6/3 -> Product26/3, Product30/1
  Demux6/4 -> Product16/2
  Demux6/5 -> Product30/2
  Product27/1 -> Sum19/1
  Sum19/1 -> I Controller5/1
  Delay10/1 -> Sum19/2
  I Controller5/1 -> Delay10/1, Delay11/1
  Product17/1 -> Cp10/1
  I7 Phase test step/1 -> Product25/1
  Sum17/1 -> Product24/2
  "I7 Phase init "/1 -> Sum17/3
  Product25/1 -> Sum17/1
  Mask6/1 -> Product25/4, Product17/1
  Cp10/1 -> I Controller5/Trigger
  Delay11/1 -> Sum17/2
  I7 Phase Step/1 -> Product27/3
  Demux7/1 -> Product24/1
  Demux7/2 -> Product25/2
  Demux7/3 -> Product25/3, Product27/1
  Demux7/4 -> Product17/2
  Demux7/5 -> Product27/2
  Product23/1 -> Sum18/1
  Sum18/1 -> I Controller6/1
  Delay12/1 -> Sum18/2
  I Controller6/1 -> Delay12/1, Delay16/1
  Product28/1 -> Cp11/1
  I9 test step/1 -> Product21/1
  Sum24/1 -> Product31/2
  "I9 init "/1 -> Sum24/3
  Product21/1 -> Sum24/1
  Mask7/1 -> Product21/4, Product28/1
  Cp11/1 -> I Controller6/Trigger
  Delay16/1 -> Sum24/2
  I9 Step/1 -> Product23/3
  Demux8/1 -> Product31/1
  Demux8/2 -> Product21/2
  Demux8/3 -> Product21/3, Product23/1
  Demux8/4 -> Product28/2
  Demux8/5 -> Product23/2
  Product22/1 -> Sum23/1
  Sum23/1 -> I Controller7/1
  Delay14/1 -> Sum23/2
  I Controller7/1 -> Delay14/1, Delay15/1
  Product29/1 -> Cp12/1
  I9 Phase test step/1 -> Product19/1
  Sum20/1 -> Product18/2
  "I9 Phase init "/1 -> Sum20/3
  Product19/1 -> Sum20/1
  Mask8/1 -> Product19/4, Product29/1
  Cp12/1 -> I Controller7/Trigger
  Delay15/1 -> Sum20/2
  I9 Phase Step/1 -> Product22/3
  Demux9/1 -> Product18/1
  Demux9/2 -> Product19/2
  Demux9/3 -> Product19/3, Product22/1
  Demux9/4 -> Product29/2
  Demux9/5 -> Product22/2
  Product31/1 -> I9/1, To File8/1
  Product18/1 -> Phase I9/1, To File9/1
  Product24/1 -> Phase I7/1, To File7/1
  x23/1 -> Sum4/3
  x24/1 -> Sum4/4
  Product39/1 -> Sum28/1
  Sum28/1 -> I Controller8/1
  Delay20/1 -> Sum28/2
  I Controller8/1 -> Delay20/1, Delay19/1
  Product32/1 -> Cp14/1
  I11 test step/1 -> Product37/1
  Product34/1 -> I11/1, To File10/1
  Sum27/1 -> Product34/2
  "I11 init "/1 -> Sum27/3
  Product37/1 -> Sum27/1
  Mask1/1 -> Product37/4, Product32/1
  Cp14/1 -> I Controller8/Trigger
  Delay19/1 -> Sum27/2
  I11 Step/1 -> Product39/3
  Demux10/1 -> Product34/1
  Demux10/2 -> Product37/2
  Demux10/3 -> Product37/3, Product39/1
  Demux10/4 -> Product32/2
  Demux10/5 -> Product39/2
  Product38/1 -> Sum26/1
  Sum26/1 -> I Controller9/1
  Delay17/1 -> Sum26/2
  I Controller9/1 -> Delay17/1, Delay18/1
  Product33/1 -> Cp13/1
  I11 Phase test step/1 -> Product36/1
  Sum25/1 -> Product35/2
  I11 Phase init 1/1 -> Sum25/3
  Product36/1 -> Sum25/1
  Mask9/1 -> Product36/4, Product33/1
  Cp13/1 -> I Controller9/Trigger
  Delay18/1 -> Sum25/2
  I11 Phase Step/1 -> Product38/3
  Demux11/1 -> Product35/1
  Demux11/2 -> Product36/2
  Demux11/3 -> Product36/3, Product38/1
  Demux11/4 -> Product33/2
  Demux11/5 -> Product38/2
  Product35/1 -> Phase I11/1, To File11/1
  SP U11/1 -> Sum29/2
  x1/1 -> Sum4/5
  Sum29/1 -> x1/1
  Demux1/5 -> Sum29/1
  Gain2/1 -> Mux1/5
  Delay8/1 -> Mux1/3
  Delay4/1 -> Sum5/3
  "I3 init "/1 -> Sum5/2
  Sign/1 -> Sum6/1
  Sign1/1 -> Sum6/2
  Delay/1 -> Sum/2
  Product8/1 -> Sum/1

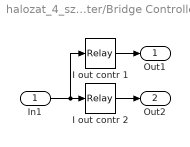
== system halozat_4_szet/Grid Synchronized Inverter/Bridge Controller ==
  In1 : Inport
  I out contr 1 : Relay  OnSwitchValue=0.1  OffSwitchValue=-0.1  OnOutputValue=10  ZeroCross=off  SampleTime=1e-4
  I out contr 2 : Relay  OnSwitchValue=0.1  OffSwitchValue=-0.1  OnOutputValue=0  OffOutputValue=10  ZeroCross=off  SampleTime=1e-4
  Out1 : Outport
  Out2 : Outport  Port=2
  wires:
  In1/1 -> I out contr 1/1, I out contr 2/1
  I out contr 1/1 -> Out1/1
  I out contr 2/1 -> Out2/1

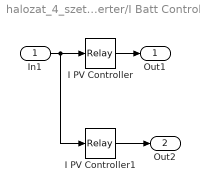
== system halozat_4_szet/Grid Synchronized Inverter/I Batt Controller ==
  In1 : Inport
  I PV Controller : Relay  OnSwitchValue=0.01  OffSwitchValue=-0.01  ZeroCross=off  SampleTime=1e-4
  I PV Controller1 : Relay  OnSwitchValue=0.01  OffSwitchValue=-0.01  OnOutputValue=0  OffOutputValue=1  ZeroCross=off  SampleTime=1e-4
  Out1 : Outport
  Out2 : Outport  Port=2
  wires:
  In1/1 -> I PV Controller/1, I PV Controller1/1
  I PV Controller/1 -> Out1/1
  I PV Controller1/1 -> Out2/1

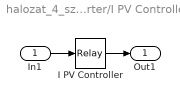
== system halozat_4_szet/Grid Synchronized Inverter/I PV Controller ==
  In1 : Inport
  I PV Controller : Relay  OnSwitchValue=0.01  OffSwitchValue=-0.01  ZeroCross=off  SampleTime=1e-4
  Out1 : Outport
  wires:
  In1/1 -> I PV Controller/1
  I PV Controller/1 -> Out1/1

== system halozat_4_szet/Grid Synchronized Inverter/I_base phase controller ==
  U_connect : Inport
  Base phase : Constant  Value=0
  I_base phase : Outport
  wires:
  Base phase/1 -> I_base phase/1

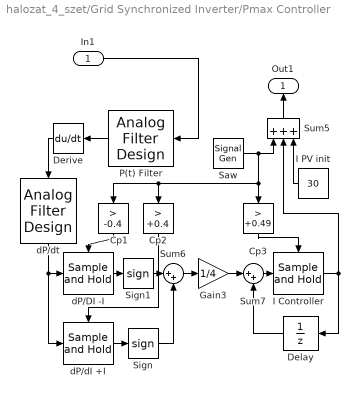
== system halozat_4_szet/Grid Synchronized Inverter/Pmax Controller ==
  In1 : Inport
  Cp1 : simulink/Logic and Bit Operations/Compare To Constant  relop=>  const=-0.4  OutDataTypeStr=uint8  ZeroCross=off
  Cp2 : simulink/Logic and Bit Operations/Compare To Constant  relop=>  const=+0.4  OutDataTypeStr=uint8  ZeroCross=off
  Cp3 : simulink/Logic and Bit Operations/Compare To Constant  relop=>  const=+0.49  OutDataTypeStr=uint8  ZeroCross=off
  Delay : UnitDelay  SampleTime=0.01
  Derive : Derivative
  Gain3 : Gain  Gain=1/4
  I Controller : dspsigops/Sample and Hold  trig=Rising edge  initCond=0  latchinput=off
  "I PV init " : Constant  Value=30
  P(t) Filter : dsparch4/Analog Filter Design  method=Butterworth  filttype=Lowpass  N=1  Wlo=628  Whi=80  Rp=2  Rs=40
  Saw : SignalGenerator  WaveForm=sawtooth  Amplitude=-0.5  Frequency=10
  Sign : Signum
  Sign1 : Signum
  Sum5 : Sum  Inputs=+++
  Sum6 : Sum  Inputs=|++
  Sum7 : Sum  Inputs=|++
  dP/DI -I : dspsigops/Sample and Hold  trig=Rising edge  initCond=0  latchinput=off
  dP/dI +I : dspsigops/Sample and Hold  trig=Rising edge  initCond=0  latchinput=off
  "dP/dt " : dsparch4/Analog Filter Design  method=Butterworth  filttype=Lowpass  N=8  Wlo=6280  Whi=80  Rp=2  Rs=40
  Out1 : Outport
  wires:
  P(t) Filter/1 -> Derive/1
  I Controller/1 -> Sum5/2, Delay/1
  "I PV init "/1 -> Sum5/3
  Sign1/1 -> Sum6/1
  dP/DI -I/1 -> Sign1/1
  Sign/1 -> Sum6/2
  dP/dI +I/1 -> Sign/1
  Delay/1 -> Sum7/2
  Saw/1 -> Sum5/1, Cp3/1, Cp2/1, Cp1/1
  Cp3/1 -> I Controller/Trigger
  Sum7/1 -> I Controller/1
  Gain3/1 -> Sum7/1
  Sum6/1 -> Gain3/1
  Cp2/1 -> dP/dI +I/Trigger
  Cp1/1 -> dP/DI -I/Trigger
  "dP/dt "/1 -> dP/DI -I/1, dP/dI +I/1
  Derive/1 -> "dP/dt "/1
  Sum5/1 -> Out1/1
  In1/1 -> P(t) Filter/1

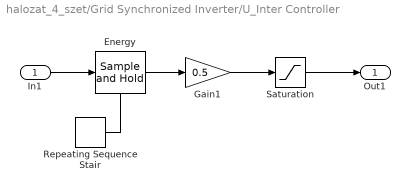
== system halozat_4_szet/Grid Synchronized Inverter/U_Inter Controller ==
  In1 : Inport
  Energy : dspsigops/Sample and Hold  trig=Rising edge  initCond=18  latchinput=off
  Gain1 : Gain  Gain=0.5
  Repeating Sequence Stair : simulink/Sources/Repeating Sequence Stair  OutValues=[ 1 0 ]  tsamp=0.01  OutMin=[]  OutMax=[]  OutDataTypeStr=float('double')  OutputDataTypeScalingMode=Specify via dialog  OutDataType=float('double')  ConRadixGroup=Best Precision: Vector-wise  OutScaling=2^-12
  Saturation : Saturate  UpperLimit=50  LowerLimit=-50
  Out1 : Outport
  wires:
  Gain1/1 -> Saturation/1
  Saturation/1 -> Out1/1
  In1/1 -> Energy/1
  Energy/1 -> Gain1/1
  Repeating Sequence Stair/1 -> Energy/Trigger
